simulink model "sampleModel1000"  (R2022a)
settings: Solver=VariableStepAuto  StartTime=0.0  StopTime=10.0  RelTol=1e-3
undefined symbols (not defined in the file): DiscIntNeverNeededParam, magnitude, Newton, Raphson
libraries: simulink x216, slpidlib x76
(part 2 of 10)

== system sampleModel1000/cfblk134 ==
  cfblk1 : Inport
  cfblk10 : Delay  SampleTime=1
  cfblk3 : simulink/Discrete/Transfer Fcn First Order  PoleZ=0.95  ICPrevOutput=0.0  DoSatur=off
  cfblk4 : DiscreteFir  SampleTime=1
  cfblk5 : slpidlib/PID Controller (2DOF)  Controller=PID  Form=Parallel  TimeDomain=Discrete-time  UseExternalTs=off  SampleTime=1  IntegratorMethod=Forward Euler  FilterMethod=Forward Euler  ControllerParametersSource=internal  P=1  I=1  UseKiTs=off  D=0  N=100  UseFilter=on  b=1  c=1  TunerSelectOption=Transfer Function Based (PID Tuner App)  InitialConditionSource=internal  InitialConditionForIntegrator=0  InitialConditionForFilter=0  DifferentiatorICPrevScaledInput=0  ExternalReset=none  TrackingMode=off  Kt=1  LimitOutput=off  SatLimitsSource=internal  UpperSaturationLimit=inf  LowerSaturationLimit=-inf  LinearizeAsGain=off  AntiWindupMode=none  Kb=1  POutMin=[]  POutMax=[]  IOutMin=[]  IOutMax=[]  DOutMin=[]  DOutMax=[]  NOutMin=[]  NOutMax=[]  bOutMin=[]  bOutMax=[]  cOutMin=[]  cOutMax=[]  SumOutMin=[]  SumOutMax=[]  SaturationOutMin=[]  SaturationOutMax=[]  PParamMin=[]  PParamMax=[]  IParamMin=[]  IParamMax=[]  DParamMin=[]  DParamMax=[]  NParamMin=[]  NParamMax=[]  bParamMin=[]  bParamMax=[]  cParamMin=[]  cParamMax=[]  KbParamMin=[]  KbParamMax=[]  KtParamMin=[]  KtParamMax=[]  KbOutMin=[]  KbOutMax=[]  KtOutMin=[]  KtOutMax=[]  IntegratorOutMin=[]  IntegratorOutMax=[]  FilterOutMin=[]  FilterOutMax=[]  SumI1OutMin=[]  SumI1OutMax=[]  SumI2OutMin=[]  SumI2OutMax=[]  SumI3OutMin=[]  SumI3OutMax=[]  SumI4OutMin=[]  SumI4OutMax=[]  SumDOutMin=[]  SumDOutMax=[]  Sum1OutMin=[]  Sum1OutMax=[]  Sum2OutMin=[]  Sum2OutMax=[]  Sum3OutMin=[]  Sum3OutMax=[]  DifferentiatorOutMin=[]  DifferentiatorOutMax=[]  FilterDiffOutCoefMin=[]  FilterDiffOutCoefMax=[]  ReciprocalOutMin=[]  ReciprocalOutMax=[]  SumDenOutMin=[]  SumDenOutMax=[]  SumNumOutMin=[]  SumNumOutMax=[]  DivideOutMin=[]  DivideOutMax=[]  UdiffTsProdOutMin=[]  UdiffTsProdOutMax=[]  NTsProdOutMin=[]  NTsProdOutMax=[]  UintegralTsProdOutMin=[]  UintegralTsProdOutMax=[]  UngainTsProdOutMin=[]  UngainTsProdOutMax=[]  IntegratorContinuousStateAttributes=''  IntegratorStateMustResolveToSignalObject=off  IntegratorRTWStateStorageClass=Auto  FilterContinuousStateAttributes=''  FilterStateMustResolveToSignalObject=off  FilterRTWStateStorageClass=Auto  ParallelPVariant=InternalParameters  IdealPVariant=Disabled  IVariant=InternalParameters  DVariant=InternalParameters  bVariant=InternalParameters  cVariant=InternalParameters  IntegratorVariant=Discrete  SatVariant=Disabled  AWVariant=Passthrough  PCopyVariant=Disabled  TRVariant=Disabled  FdbkBlocksVariant=Forward  IdealPFdbkVariant=Disabled  SatFdbkVariant=Disabled  DerivativeFilterVariant=ForwardEulerFilter  NVariant=InternalParameters  NCopyVariant=Disabled  FilterICVariant=InternalICsFilter  IntegratorICVariant=InternalICs  ExternalResetVariant=Disabled  TRSumVariant=Passthrough  SumFdbkVariant=Disabled  SumVariant=Sum_PID  TsampFilterVariant=InternalTs  TsampNgainVariant=Passthrough  TsampIntegralVariant=Passthrough  ExternalSaturationOutDataTypeStr=Inherit: Same as second input
      settings: SourceProductBaseCode=SL
  cfblk6 : DotProduct  OutDataTypeStr=Inherit: Inherit via internal rule
  cfblk7 : Product
  cfblk9 : Delay  SampleTime=1
  cfblk2 : Outport
  cfblk8 : Outport  Port=2
  wires:
  cfblk7/1 -> cfblk3/1, cfblk4/1
  cfblk5/1 -> cfblk6/1, cfblk2/1
  cfblk1/1 -> cfblk5/2
  cfblk6/1 -> cfblk7/1, cfblk7/2, cfblk8/1
  cfblk3/1 -> cfblk9/1
  cfblk9/1 -> cfblk5/1
  cfblk4/1 -> cfblk10/1
  cfblk10/1 -> cfblk6/2

== system sampleModel1000/cfblk135 ==
  cfblk1 : Inport
  cfblk15 : Inport  Port=2
  cfblk16 : Inport  Port=3
  cfblk10 : Sqrt
  cfblk11 : Constant  Value=[-838674796.182005]  SampleTime=1
  cfblk12 : Subsystem
  cfblk13 : Subsystem
  cfblk14 : Subsystem
  cfblk17 : Delay  SampleTime=1
  cfblk3 : DiscreteStateSpace
  cfblk4 : Delay  SampleTime=1
  cfblk5 : DiscreteZeroPole  Poles=[0 0.5]  Gain=1
  cfblk6 : Math  Operator=transpose
  cfblk7 : ComplexToRealImag
  cfblk8 : Product
  cfblk9 : simulink/Math Operations/Slider Gain  gain=1  low=0  high=2
  cfblk2 : Outport
  wires:
  cfblk5/1 -> cfblk3/1
  cfblk1/1 -> cfblk6/1
  cfblk11/1 -> cfblk14/1(cfblk1)
  cfblk15/1 -> cfblk10/1
  cfblk16/1 -> cfblk7/1
  cfblk8/1 -> cfblk12/1(cfblk1)
  cfblk12/1(cfblk2) -> cfblk9/1
  cfblk9/1 -> cfblk14/2(cfblk9)
  cfblk4/1 -> cfblk5/1
  cfblk7/1 -> cfblk14/3(cfblk10)
  cfblk13/1(cfblk2) -> cfblk4/1
  cfblk3/1 -> cfblk2/1
  cfblk10/1 -> cfblk8/2
  cfblk7/2 -> cfblk13/1(cfblk1)
  cfblk13/2(cfblk15) -> cfblk14/4(cfblk11)
  cfblk12/2(cfblk14) -> cfblk17/1
  cfblk17/1 -> cfblk8/1

== system sampleModel1000/cfblk136 ==
  cfblk1 : Inport
  cfblk9 : Inport  Port=2
  cfblk10 : Inport  Port=3
  cfblk12 : Delay  SampleTime=1
  cfblk13 : Delay  SampleTime=1
  cfblk3 : slpidlib/PID Controller  Controller=PID  Form=Parallel  TimeDomain=Discrete-time  UseExternalTs=off  SampleTime=1  IntegratorMethod=Forward Euler  FilterMethod=Forward Euler  ControllerParametersSource=internal  P=1  I=1  UseKiTs=off  D=0  N=100  UseFilter=on  TunerSelectOption=Transfer Function Based (PID Tuner App)  InitialConditionSource=internal  InitialConditionForIntegrator=0  InitialConditionForFilter=0  DifferentiatorICPrevScaledInput=0  ExternalReset=none  TrackingMode=off  Kt=1  LimitOutput=off  SatLimitsSource=internal  UpperSaturationLimit=inf  LowerSaturationLimit=-inf  LinearizeAsGain=off  AntiWindupMode=none  Kb=1  POutMin=[]  POutMax=[]  IOutMin=[]  IOutMax=[]  DOutMin=[]  DOutMax=[]  NOutMin=[]  NOutMax=[]  SumOutMin=[]  SumOutMax=[]  SaturationOutMin=[]  SaturationOutMax=[]  PParamMin=[]  PParamMax=[]  IParamMin=[]  IParamMax=[]  DParamMin=[]  DParamMax=[]  NParamMin=[]  NParamMax=[]  KbParamMin=[]  KbParamMax=[]  KtParamMin=[]  KtParamMax=[]  KbOutMin=[]  KbOutMax=[]  KtOutMin=[]  KtOutMax=[]  IntegratorOutMin=[]  IntegratorOutMax=[]  FilterOutMin=[]  FilterOutMax=[]  SumI1OutMin=[]  SumI1OutMax=[]  SumI2OutMin=[]  SumI2OutMax=[]  SumI3OutMin=[]  SumI3OutMax=[]  SumI4OutMin=[]  SumI4OutMax=[]  SumDOutMin=[]  SumDOutMax=[]  DifferentiatorOutMin=[]  DifferentiatorOutMax=[]  FilterDiffOutCoefMin=[]  FilterDiffOutCoefMax=[]  ReciprocalOutMin=[]  ReciprocalOutMax=[]  SumDenOutMin=[]  SumDenOutMax=[]  SumNumOutMin=[]  SumNumOutMax=[]  DivideOutMin=[]  DivideOutMax=[]  UdiffTsProdOutMin=[]  UdiffTsProdOutMax=[]  NTsProdOutMin=[]  NTsProdOutMax=[]  UintegralTsProdOutMin=[]  UintegralTsProdOutMax=[]  UngainTsProdOutMin=[]  UngainTsProdOutMax=[]  IntegratorContinuousStateAttributes=''  IntegratorStateMustResolveToSignalObject=off  IntegratorRTWStateStorageClass=Auto  FilterContinuousStateAttributes=''  FilterStateMustResolveToSignalObject=off  FilterRTWStateStorageClass=Auto  ParallelPVariant=InternalParameters  IdealPVariant=Disabled  IVariant=InternalParameters  DVariant=InternalParameters  IntegratorVariant=Discrete  SatVariant=Disabled  AWVariant=Passthrough  PCopyVariant=Disabled  TRVariant=Disabled  FdbkBlocksVariant=Forward  IdealPFdbkVariant=Disabled  SatFdbkVariant=Disabled  DerivativeFilterVariant=ForwardEulerFilter  NVariant=InternalParameters  NCopyVariant=Disabled  FilterICVariant=InternalICsFilter  IntegratorICVariant=InternalICs  ExternalResetVariant=Disabled  TRSumVariant=Passthrough  SumFdbkVariant=Disabled  SumVariant=Sum_PID  TsampFilterVariant=InternalTs  TsampNgainVariant=Passthrough  TsampIntegralVariant=Passthrough  ExternalSaturationOutDataTypeStr=Inherit: Same as second input  aMode=0
  cfblk4 : slpidlib/PID Controller  Controller=PID  Form=Parallel  TimeDomain=Discrete-time  UseExternalTs=off  SampleTime=1  IntegratorMethod=Forward Euler  FilterMethod=Forward Euler  ControllerParametersSource=internal  P=1  I=1  UseKiTs=off  D=0  N=100  UseFilter=on  TunerSelectOption=Transfer Function Based (PID Tuner App)  InitialConditionSource=internal  InitialConditionForIntegrator=0  InitialConditionForFilter=0  DifferentiatorICPrevScaledInput=0  ExternalReset=none  TrackingMode=off  Kt=1  LimitOutput=off  SatLimitsSource=internal  UpperSaturationLimit=inf  LowerSaturationLimit=-inf  LinearizeAsGain=off  AntiWindupMode=none  Kb=1  POutMin=[]  POutMax=[]  IOutMin=[]  IOutMax=[]  DOutMin=[]  DOutMax=[]  NOutMin=[]  NOutMax=[]  SumOutMin=[]  SumOutMax=[]  SaturationOutMin=[]  SaturationOutMax=[]  PParamMin=[]  PParamMax=[]  IParamMin=[]  IParamMax=[]  DParamMin=[]  DParamMax=[]  NParamMin=[]  NParamMax=[]  KbParamMin=[]  KbParamMax=[]  KtParamMin=[]  KtParamMax=[]  KbOutMin=[]  KbOutMax=[]  KtOutMin=[]  KtOutMax=[]  IntegratorOutMin=[]  IntegratorOutMax=[]  FilterOutMin=[]  FilterOutMax=[]  SumI1OutMin=[]  SumI1OutMax=[]  SumI2OutMin=[]  SumI2OutMax=[]  SumI3OutMin=[]  SumI3OutMax=[]  SumI4OutMin=[]  SumI4OutMax=[]  SumDOutMin=[]  SumDOutMax=[]  DifferentiatorOutMin=[]  DifferentiatorOutMax=[]  FilterDiffOutCoefMin=[]  FilterDiffOutCoefMax=[]  ReciprocalOutMin=[]  ReciprocalOutMax=[]  SumDenOutMin=[]  SumDenOutMax=[]  SumNumOutMin=[]  SumNumOutMax=[]  DivideOutMin=[]  DivideOutMax=[]  UdiffTsProdOutMin=[]  UdiffTsProdOutMax=[]  NTsProdOutMin=[]  NTsProdOutMax=[]  UintegralTsProdOutMin=[]  UintegralTsProdOutMax=[]  UngainTsProdOutMin=[]  UngainTsProdOutMax=[]  IntegratorContinuousStateAttributes=''  IntegratorStateMustResolveToSignalObject=off  IntegratorRTWStateStorageClass=Auto  FilterContinuousStateAttributes=''  FilterStateMustResolveToSignalObject=off  FilterRTWStateStorageClass=Auto  ParallelPVariant=InternalParameters  IdealPVariant=Disabled  IVariant=InternalParameters  DVariant=InternalParameters  IntegratorVariant=Discrete  SatVariant=Disabled  AWVariant=Passthrough  PCopyVariant=Disabled  TRVariant=Disabled  FdbkBlocksVariant=Forward  IdealPFdbkVariant=Disabled  SatFdbkVariant=Disabled  DerivativeFilterVariant=ForwardEulerFilter  NVariant=InternalParameters  NCopyVariant=Disabled  FilterICVariant=InternalICsFilter  IntegratorICVariant=InternalICs  ExternalResetVariant=Disabled  TRSumVariant=Passthrough  SumFdbkVariant=Disabled  SumVariant=Sum_PID  TsampFilterVariant=InternalTs  TsampNgainVariant=Passthrough  TsampIntegralVariant=Passthrough  ExternalSaturationOutDataTypeStr=Inherit: Same as second input  aMode=0
  cfblk5 : MinMax  Function=max  Inputs=2
  cfblk6 : Subsystem
  cfblk7 : Subsystem
  cfblk8 : Subsystem
  cfblk2 : Outport
  cfblk11 : Outport  Port=2
  wires:
  cfblk7/1(cfblk2) -> cfblk6/1(cfblk1)
  cfblk8/1(cfblk2) -> cfblk3/1
  cfblk10/1 -> cfblk4/1, cfblk8/4(cfblk9)
  cfblk8/2(cfblk12) -> cfblk2/1
  cfblk1/1 -> cfblk11/1, cfblk7/3(cfblk6)
  cfblk9/1 -> cfblk7/1(cfblk1)
  cfblk4/1 -> cfblk6/2(cfblk10)
  cfblk6/1(cfblk2) -> cfblk8/2(cfblk7), cfblk5/2, cfblk8/6(cfblk11)
  cfblk7/2(cfblk7) -> cfblk8/3(cfblk8), cfblk8/5(cfblk10)
  cfblk3/1 -> cfblk5/1, cfblk13/1
  cfblk5/1 -> cfblk12/1
  cfblk12/1 -> cfblk8/1(cfblk1)
  cfblk13/1 -> cfblk7/2(cfblk5)

== system sampleModel1000/cfblk137 ==
  cfblk1 : Inport
  cfblk13 : Inport  Port=2
  cfblk10 : Constant  Value=[-152590249.927515]  SampleTime=1
  cfblk11 : Constant  Value=[315107042.887950]  SampleTime=1
  cfblk12 : Subsystem
  cfblk3 : DiscreteFir  SampleTime=1
  cfblk4 : DiscreteStateSpace
  cfblk5 : Assignment  DiagnosticForDimensions=Warning  IndexOptions=Index vector (dialog)  Indices=1  OutputSizes=1
  cfblk6 : Sqrt  Operator=rSqrt  AlgorithmType=Newton-Raphson
  cfblk7 : Abs  SaturateOnIntegerOverflow=off
  cfblk8 : UnaryMinus
  cfblk9 : Signum
  cfblk2 : Outport
  cfblk14 : Outport  Port=2
  cfblk15 : Outport  Port=3
  wires:
  cfblk9/1 -> cfblk6/1
  cfblk13/1 -> cfblk12/1(cfblk1)
  cfblk8/1 -> cfblk5/1
  cfblk1/1 -> cfblk12/2(cfblk8)
  cfblk3/1 -> cfblk4/1
  cfblk4/1 -> cfblk2/1
  cfblk11/1 -> cfblk15/1
  cfblk10/1 -> cfblk7/1
  cfblk7/1 -> cfblk8/1
  cfblk6/1 -> cfblk5/2
  cfblk5/1 -> cfblk14/1
  cfblk12/1(cfblk2) -> cfblk3/1
  cfblk12/2(cfblk9) -> cfblk9/1

== system sampleModel1000/cfblk138 ==
  cfblk1 : Inport
  cfblk11 : Inport  Port=2
  cfblk10 : Subsystem
  cfblk3 : Delay  DelayLengthSource=Input port  SampleTime=1
      settings: InputPortMap=u0,p1
  cfblk4 : simulink/Discrete/Transfer Fcn Lead or Lag  PoleZ=0.95  ZeroZ=0.75  ICPrevOutput=0.0  ICPrevInput=0.0  DoSatur=off
      settings: SourceProductBaseCode=SL
  cfblk5 : ComplexToMagnitudeAngle
  cfblk6 : Trigonometry
  cfblk7 : Constant  Value=[211032908.922208]  SampleTime=1
  cfblk8 : Constant  Value=[325607232.572119]  SampleTime=1
  cfblk9 : Constant  Value=[286958174.606833]  SampleTime=1
  cfblk2 : Outport
  cfblk12 : Outport  Port=2
  wires:
  cfblk9/1 -> cfblk2/1
  cfblk10/1(cfblk2) -> cfblk12/1
  cfblk8/1 -> cfblk4/1
  cfblk11/1 -> cfblk3/1
  cfblk3/1 -> cfblk6/1
  cfblk5/1 -> cfblk3/2
  cfblk4/1 -> cfblk5/1
  cfblk7/1 -> cfblk10/1(cfblk1)
  cfblk1/1 -> cfblk10/2(cfblk13)
  cfblk6/1 -> cfblk10/3(cfblk14)

== system sampleModel1000/cfblk139 ==
  cfblk1 : Inport
  cfblk14 : Inport  Port=2
  cfblk15 : Inport  Port=3
  cfblk10 : Constant  Value=[730462996.486864]  SampleTime=1
  cfblk11 : Subsystem
  cfblk12 : Subsystem
  cfblk13 : Subsystem
  cfblk16 : Delay  SampleTime=1
  cfblk17 : Delay  SampleTime=1
  cfblk3 : slpidlib/PID Controller  Controller=PID  Form=Parallel  TimeDomain=Discrete-time  UseExternalTs=off  SampleTime=1  IntegratorMethod=Forward Euler  FilterMethod=Forward Euler  ControllerParametersSource=internal  P=1  I=1  UseKiTs=off  D=0  N=100  UseFilter=on  TunerSelectOption=Transfer Function Based (PID Tuner App)  InitialConditionSource=internal  InitialConditionForIntegrator=0  InitialConditionForFilter=0  DifferentiatorICPrevScaledInput=0  ExternalReset=none  TrackingMode=off  Kt=1  LimitOutput=off  SatLimitsSource=internal  UpperSaturationLimit=inf  LowerSaturationLimit=-inf  LinearizeAsGain=off  AntiWindupMode=none  Kb=1  POutMin=[]  POutMax=[]  IOutMin=[]  IOutMax=[]  DOutMin=[]  DOutMax=[]  NOutMin=[]  NOutMax=[]  SumOutMin=[]  SumOutMax=[]  SaturationOutMin=[]  SaturationOutMax=[]  PParamMin=[]  PParamMax=[]  IParamMin=[]  IParamMax=[]  DParamMin=[]  DParamMax=[]  NParamMin=[]  NParamMax=[]  KbParamMin=[]  KbParamMax=[]  KtParamMin=[]  KtParamMax=[]  KbOutMin=[]  KbOutMax=[]  KtOutMin=[]  KtOutMax=[]  IntegratorOutMin=[]  IntegratorOutMax=[]  FilterOutMin=[]  FilterOutMax=[]  SumI1OutMin=[]  SumI1OutMax=[]  SumI2OutMin=[]  SumI2OutMax=[]  SumI3OutMin=[]  SumI3OutMax=[]  SumI4OutMin=[]  SumI4OutMax=[]  SumDOutMin=[]  SumDOutMax=[]  DifferentiatorOutMin=[]  DifferentiatorOutMax=[]  FilterDiffOutCoefMin=[]  FilterDiffOutCoefMax=[]  ReciprocalOutMin=[]  ReciprocalOutMax=[]  SumDenOutMin=[]  SumDenOutMax=[]  SumNumOutMin=[]  SumNumOutMax=[]  DivideOutMin=[]  DivideOutMax=[]  UdiffTsProdOutMin=[]  UdiffTsProdOutMax=[]  NTsProdOutMin=[]  NTsProdOutMax=[]  UintegralTsProdOutMin=[]  UintegralTsProdOutMax=[]  UngainTsProdOutMin=[]  UngainTsProdOutMax=[]  IntegratorContinuousStateAttributes=''  IntegratorStateMustResolveToSignalObject=off  IntegratorRTWStateStorageClass=Auto  FilterContinuousStateAttributes=''  FilterStateMustResolveToSignalObject=off  FilterRTWStateStorageClass=Auto  ParallelPVariant=InternalParameters  IdealPVariant=Disabled  IVariant=InternalParameters  DVariant=InternalParameters  IntegratorVariant=Discrete  SatVariant=Disabled  AWVariant=Passthrough  PCopyVariant=Disabled  TRVariant=Disabled  FdbkBlocksVariant=Forward  IdealPFdbkVariant=Disabled  SatFdbkVariant=Disabled  DerivativeFilterVariant=ForwardEulerFilter  NVariant=InternalParameters  NCopyVariant=Disabled  FilterICVariant=InternalICsFilter  IntegratorICVariant=InternalICs  ExternalResetVariant=Disabled  TRSumVariant=Passthrough  SumFdbkVariant=Disabled  SumVariant=Sum_PID  TsampFilterVariant=InternalTs  TsampNgainVariant=Passthrough  TsampIntegralVariant=Passthrough  ExternalSaturationOutDataTypeStr=Inherit: Same as second input  aMode=0
  cfblk4 : DiscreteTransferFcn  SampleTime=1
  cfblk5 : UnitDelay  HasFrameUpgradeWarning=on
  cfblk6 : simulink/Math Operations/MinMax Running Resettable  Function=min  vinit=0.0
  cfblk7 : PermuteDimensions
  cfblk8 : UnaryMinus
  cfblk9 : MinMax  Inputs=3
  cfblk2 : Outport
  wires:
  cfblk3/1 -> cfblk5/1
  cfblk9/1 -> cfblk7/1
  cfblk7/1 -> cfblk6/1
  cfblk8/1 -> cfblk9/1
  cfblk4/1 -> cfblk12/1(cfblk1)
  cfblk14/1 -> cfblk9/2, cfblk11/3(cfblk10)
  cfblk5/1 -> cfblk12/2(cfblk10), cfblk4/1
  cfblk10/1 -> cfblk3/1
  cfblk12/1(cfblk2) -> cfblk8/1
  cfblk15/1 -> cfblk11/1(cfblk1)
  cfblk1/1 -> cfblk12/3(cfblk11), cfblk13/2(cfblk10), cfblk12/4(cfblk12), cfblk13/3(cfblk11), cfblk11/4(cfblk11)
  cfblk13/1(cfblk2) -> cfblk11/2(cfblk9), cfblk12/5(cfblk13)
  cfblk12/2(cfblk14) -> cfblk6/2
  cfblk12/3(cfblk15) -> cfblk2/1
  cfblk6/1 -> cfblk16/1
  cfblk16/1 -> cfblk9/3
  cfblk11/1(cfblk2) -> cfblk17/1
  cfblk17/1 -> cfblk13/1(cfblk1)

== system sampleModel1000/cfblk140 ==
  cfblk1 : Inport
  cfblk8 : Inport  Port=2
  cfblk{9..13} (5 alike) : Delay  SampleTime=1
  cfblk3 : simulink/Discrete/Transfer Fcn Real Zero  ZeroZ=0.75  ICPrevInput=0.0  DoSatur=off
      settings: SourceProductBaseCode=SL
  cfblk4 : Delay  DelayLengthSource=Input port  SampleTime=1
      settings: InputPortMap=u0,p1
  cfblk5 : UnitDelay  HasFrameUpgradeWarning=on
  cfblk6 : Subsystem
  cfblk7 : Subsystem
  cfblk2 : Outport
  wires:
  cfblk5/1 -> cfblk6/1(cfblk1)
  cfblk8/1 -> cfblk5/1
  cfblk1/1 -> cfblk7/2(cfblk15), cfblk4/2
  cfblk6/1(cfblk2) -> cfblk3/1
  cfblk3/1 -> cfblk2/1, cfblk4/1, cfblk10/1, cfblk11/1, cfblk12/1
  cfblk7/1(cfblk2) -> cfblk6/2(cfblk8)
  cfblk4/1 -> cfblk9/1
  cfblk9/1 -> cfblk7/1(cfblk1)
  cfblk10/1 -> cfblk6/3(cfblk9)
  cfblk11/1 -> cfblk6/4(cfblk10)
  cfblk12/1 -> cfblk7/4(cfblk17)
  cfblk6/2(cfblk11) -> cfblk13/1
  cfblk13/1 -> cfblk7/3(cfblk16)

== system sampleModel1000/cfblk141 ==
  cfblk1 : Inport
  cfblk9 : Inport  Port=2
  cfblk10 : Inport  Port=3
  cfblk11 : Inport  Port=4
  cfblk3 : Delay  SampleTime=1
  cfblk4 : DiscreteZeroPole  Poles=[0 0.5]  Gain=1
  cfblk5 : Sin  TimeSource=Use external signal  SampleTime=0
  cfblk6 : Reshape
  cfblk7 : Product  Inputs=*
  cfblk8 : Subsystem
  cfblk2 : Outport
  wires:
  cfblk11/1 -> cfblk3/1
  cfblk6/1 -> cfblk4/1
  cfblk3/1 -> cfblk6/1
  cfblk7/1 -> cfblk5/1
  cfblk5/1 -> cfblk8/1(cfblk1)
  cfblk4/1 -> cfblk7/1
  cfblk9/1 -> cfblk8/2(cfblk12)
  cfblk10/1 -> cfblk8/3(cfblk13)
  cfblk8/1(cfblk2) -> cfblk2/1

== system sampleModel1000/cfblk142 ==
  cfblk1 : Inport
  cfblk10 : Subsystem
  cfblk11 : Subsystem
  cfblk12 : Subsystem
  cfblk13 : Subsystem
  cfblk{15..18} (4 alike) : Delay  SampleTime=1
  cfblk3 : DiscreteFir  SampleTime=1
  cfblk4 : simulink/Discrete/Transfer Fcn Lead or Lag  PoleZ=0.95  ZeroZ=0.75  ICPrevOutput=0.0  ICPrevInput=0.0  DoSatur=off
      settings: SourceProductBaseCode=SL
  cfblk5 : ComplexToMagnitudeAngle
  cfblk6 : Product  Inputs=**
  cfblk7 : ComplexToMagnitudeAngle
  cfblk8 : Product  Inputs=*
  cfblk9 : Constant  Value=[148580806.224860]  SampleTime=1
  cfblk2 : Outport
  cfblk14 : Outport  Port=2
  wires:
  cfblk1/1 -> cfblk10/1(cfblk1)
  cfblk6/1 -> cfblk13/3(cfblk14), cfblk18/1
  cfblk7/1 -> cfblk4/1
  cfblk10/1(cfblk2) -> cfblk8/1
  cfblk8/1 -> cfblk7/1, cfblk13/2(cfblk13)
  cfblk9/1 -> cfblk6/1
  cfblk12/1(cfblk2) -> cfblk5/1
  cfblk10/2(cfblk12) -> cfblk13/1(cfblk1), cfblk12/4(cfblk9)
  cfblk11/1(cfblk2) -> cfblk3/1
  cfblk3/1 -> cfblk15/1, cfblk16/1
  cfblk4/1 -> cfblk14/1, cfblk11/4(cfblk15)
  cfblk13/1(cfblk2) -> cfblk2/1
  cfblk7/2 -> cfblk11/2(cfblk13)
  cfblk5/2 -> cfblk6/2
  cfblk11/2(cfblk16) -> cfblk12/2(cfblk7)
  cfblk11/3(cfblk17) -> cfblk12/3(cfblk8)
  cfblk15/1 -> cfblk11/1(cfblk1)
  cfblk16/1 -> cfblk11/3(cfblk14)
  cfblk5/1 -> cfblk17/1
  cfblk17/1 -> cfblk12/1(cfblk1)
  cfblk18/1 -> cfblk10/2(cfblk11)

== system sampleModel1000/cfblk143 ==
  cfblk1 : Inport
  cfblk12 : Inport  Port=2
  cfblk10 : Constant  Value=[905866225.298065]  SampleTime=1
  cfblk11 : Subsystem
  cfblk14 : Delay  SampleTime=1
  cfblk3 : Abs  SaturateOnIntegerOverflow=off
  cfblk4 : Rounding
  cfblk5 : Sqrt  Operator=rSqrt  AlgorithmType=Newton-Raphson
  cfblk6 : Sum  Inputs=-+
  cfblk7 : Abs  SaturateOnIntegerOverflow=off
  cfblk8 : Sum  Inputs=+-
  cfblk9 : Constant  Value=[459060149.907178]  SampleTime=1
  cfblk2 : Outport
  cfblk13 : Outport  Port=2
  wires:
  cfblk1/1 -> cfblk2/1
  cfblk6/1 -> cfblk11/1(cfblk1)
  cfblk9/1 -> cfblk4/1
  cfblk7/1 -> cfblk6/1
  cfblk5/1 -> cfblk8/1
  cfblk3/1 -> cfblk7/1
  cfblk10/1 -> cfblk8/2, cfblk11/3(cfblk10)
  cfblk12/1 -> cfblk3/1
  cfblk8/1 -> cfblk13/1, cfblk14/1
  cfblk4/1 -> cfblk6/2
  cfblk11/1(cfblk2) -> cfblk5/1
  cfblk14/1 -> cfblk11/2(cfblk9)

== system sampleModel1000/cfblk144 ==
  cfblk1 : Inport
  cfblk7 : Inport  Port=2
  cfblk8 : Inport  Port=3
  cfblk3 : slpidlib/PID Controller  Controller=PID  Form=Parallel  TimeDomain=Discrete-time  UseExternalTs=off  SampleTime=1  IntegratorMethod=Forward Euler  FilterMethod=Forward Euler  ControllerParametersSource=internal  P=1  I=1  UseKiTs=off  D=0  N=100  UseFilter=on  TunerSelectOption=Transfer Function Based (PID Tuner App)  InitialConditionSource=internal  InitialConditionForIntegrator=0  InitialConditionForFilter=0  DifferentiatorICPrevScaledInput=0  ExternalReset=none  TrackingMode=off  Kt=1  LimitOutput=off  SatLimitsSource=internal  UpperSaturationLimit=inf  LowerSaturationLimit=-inf  LinearizeAsGain=off  AntiWindupMode=none  Kb=1  POutMin=[]  POutMax=[]  IOutMin=[]  IOutMax=[]  DOutMin=[]  DOutMax=[]  NOutMin=[]  NOutMax=[]  SumOutMin=[]  SumOutMax=[]  SaturationOutMin=[]  SaturationOutMax=[]  PParamMin=[]  PParamMax=[]  IParamMin=[]  IParamMax=[]  DParamMin=[]  DParamMax=[]  NParamMin=[]  NParamMax=[]  KbParamMin=[]  KbParamMax=[]  KtParamMin=[]  KtParamMax=[]  KbOutMin=[]  KbOutMax=[]  KtOutMin=[]  KtOutMax=[]  IntegratorOutMin=[]  IntegratorOutMax=[]  FilterOutMin=[]  FilterOutMax=[]  SumI1OutMin=[]  SumI1OutMax=[]  SumI2OutMin=[]  SumI2OutMax=[]  SumI3OutMin=[]  SumI3OutMax=[]  SumI4OutMin=[]  SumI4OutMax=[]  SumDOutMin=[]  SumDOutMax=[]  DifferentiatorOutMin=[]  DifferentiatorOutMax=[]  FilterDiffOutCoefMin=[]  FilterDiffOutCoefMax=[]  ReciprocalOutMin=[]  ReciprocalOutMax=[]  SumDenOutMin=[]  SumDenOutMax=[]  SumNumOutMin=[]  SumNumOutMax=[]  DivideOutMin=[]  DivideOutMax=[]  UdiffTsProdOutMin=[]  UdiffTsProdOutMax=[]  NTsProdOutMin=[]  NTsProdOutMax=[]  UintegralTsProdOutMin=[]  UintegralTsProdOutMax=[]  UngainTsProdOutMin=[]  UngainTsProdOutMax=[]  IntegratorContinuousStateAttributes=''  IntegratorStateMustResolveToSignalObject=off  IntegratorRTWStateStorageClass=Auto  FilterContinuousStateAttributes=''  FilterStateMustResolveToSignalObject=off  FilterRTWStateStorageClass=Auto  ParallelPVariant=InternalParameters  IdealPVariant=Disabled  IVariant=InternalParameters  DVariant=InternalParameters  IntegratorVariant=Discrete  SatVariant=Disabled  AWVariant=Passthrough  PCopyVariant=Disabled  TRVariant=Disabled  FdbkBlocksVariant=Forward  IdealPFdbkVariant=Disabled  SatFdbkVariant=Disabled  DerivativeFilterVariant=ForwardEulerFilter  NVariant=InternalParameters  NCopyVariant=Disabled  FilterICVariant=InternalICsFilter  IntegratorICVariant=InternalICs  ExternalResetVariant=Disabled  TRSumVariant=Passthrough  SumFdbkVariant=Disabled  SumVariant=Sum_PID  TsampFilterVariant=InternalTs  TsampNgainVariant=Passthrough  TsampIntegralVariant=Passthrough  ExternalSaturationOutDataTypeStr=Inherit: Same as second input  aMode=0
  cfblk4 : Delay  DelayLengthSource=Input port  SampleTime=1
      settings: InputPortMap=u0,p1
  cfblk5 : Gain  Gain=[419845500.922329]
  cfblk6 : Subsystem
  cfblk2 : Outport
  cfblk9 : Outport  Port=2
  wires:
  cfblk6/1(cfblk2) -> cfblk3/1
  cfblk1/1 -> cfblk5/1, cfblk6/4(cfblk14)
  cfblk3/1 -> cfblk2/1
  cfblk5/1 -> cfblk4/1, cfblk4/2, cfblk9/1
  cfblk8/1 -> cfblk6/1(cfblk1), cfblk6/5(cfblk15), cfblk6/6(cfblk16)
  cfblk7/1 -> cfblk6/2(cfblk12)
  cfblk4/1 -> cfblk6/3(cfblk13)

== system sampleModel1000/cfblk145 ==
  cfblk1 : Inport
  cfblk12 : Inport  Port=2
  cfblk13 : Inport  Port=3
  cfblk10 : Subsystem
  cfblk11 : Subsystem
  cfblk{16..19} (4 alike) : Delay  SampleTime=1
  cfblk3 : DiscreteStateSpace
  cfblk4 : ComplexToRealImag
  cfblk5 : Constant  Value=[-195042081.947706]  SampleTime=1
  cfblk6 : Constant  Value=[-214759088.337772]  SampleTime=1
  cfblk7 : Subsystem
  cfblk8 : Subsystem
  cfblk9 : Subsystem
  cfblk2 : Outport
  cfblk14 : Outport  Port=2
  cfblk15 : Outport  Port=3
  wires:
  cfblk9/1(cfblk2) -> cfblk2/1
  cfblk12/1 -> cfblk8/1(cfblk1)
  cfblk4/1 -> cfblk3/1
  cfblk9/2(cfblk12) -> cfblk8/2(cfblk7)
  cfblk13/1 -> cfblk15/1, cfblk7/5(cfblk15)
  cfblk7/1(cfblk2) -> cfblk14/1
  cfblk8/1(cfblk2) -> cfblk11/1(cfblk1)
  cfblk4/2 -> cfblk10/1(cfblk1)
  cfblk1/1 -> cfblk7/1(cfblk1), cfblk7/4(cfblk14), cfblk7/6(cfblk16)
  cfblk5/1 -> cfblk8/3(cfblk8)
  cfblk7/2(cfblk17) -> cfblk9/1(cfblk1)
  cfblk6/1 -> cfblk4/1
  cfblk3/1 -> cfblk10/2(cfblk16)
  cfblk8/2(cfblk9) -> cfblk10/3(cfblk17)
  cfblk11/1(cfblk2) -> cfblk16/1
  cfblk16/1 -> cfblk9/2(cfblk10)
  cfblk11/2(cfblk6) -> cfblk17/1
  cfblk17/1 -> cfblk7/2(cfblk12)
  cfblk11/3(cfblk7) -> cfblk18/1
  cfblk18/1 -> cfblk7/3(cfblk13)
  cfblk10/1(cfblk2) -> cfblk19/1
  cfblk19/1 -> cfblk9/3(cfblk11)

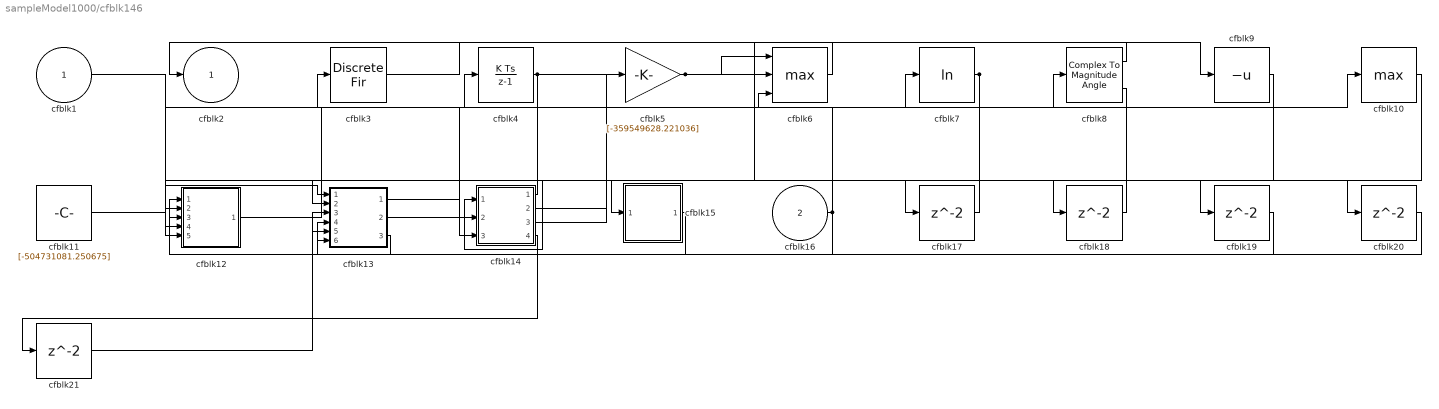
== system sampleModel1000/cfblk146 ==
  cfblk1 : Inport
  cfblk16 : Inport  Port=2
  cfblk10 : MinMax  Function=max
  cfblk11 : Constant  Value=[-504731081.250675]  SampleTime=1
  cfblk12 : Subsystem
  cfblk13 : Subsystem
  cfblk14 : Subsystem
  cfblk15 : Subsystem
  cfblk{17..21} (5 alike) : Delay  SampleTime=1
  cfblk3 : DiscreteFir  SampleTime=1
  cfblk4 : DiscreteIntegrator  ICPrevOutput=DiscIntNeverNeededParam  ICPrevScaledInput=DiscIntNeverNeededParam
  cfblk5 : Gain  Gain=[-359549628.221036]
  cfblk6 : MinMax  Function=max  Inputs=3
  cfblk7 : Math  Operator=log
  cfblk8 : ComplexToMagnitudeAngle
  cfblk9 : UnaryMinus
  cfblk2 : Outport
  wires:
  cfblk14/1(cfblk2) -> cfblk4/1
  cfblk6/1 -> cfblk2/1
  cfblk15/1(cfblk2) -> cfblk12/1(cfblk1)
  cfblk7/1 -> cfblk14/1(cfblk1), cfblk12/4(cfblk15)
  cfblk9/1 -> cfblk15/1(cfblk1)
  cfblk14/2(cfblk14) -> cfblk10/1
  cfblk10/1 -> cfblk12/2(cfblk13)
  cfblk5/1 -> cfblk6/1, cfblk19/1, cfblk20/1
  cfblk3/1 -> cfblk9/1
  cfblk12/1(cfblk2) -> cfblk8/1
  cfblk4/1 -> cfblk12/5(cfblk16), cfblk17/1
  cfblk1/1 -> cfblk13/1(cfblk1)
  cfblk16/1 -> cfblk3/1, cfblk13/4(cfblk13)
  cfblk8/1 -> cfblk6/2
  cfblk11/1 -> cfblk7/1
  cfblk13/1(cfblk2) -> cfblk6/3
  cfblk14/3(cfblk15) -> cfblk5/1
  cfblk13/2(cfblk16) -> cfblk14/3(cfblk13)
  cfblk13/3(cfblk17) -> cfblk12/3(cfblk14)
  cfblk17/1 -> cfblk14/2(cfblk12)
  cfblk8/2 -> cfblk18/1
  cfblk18/1 -> cfblk13/2(cfblk11)
  cfblk19/1 -> cfblk13/5(cfblk14)
  cfblk20/1 -> cfblk13/6(cfblk15)
  cfblk14/4(cfblk16) -> cfblk21/1
  cfblk21/1 -> cfblk13/3(cfblk12)

== system sampleModel1000/cfblk147 ==
  cfblk1 : Inport
  cfblk12 : Inport  Port=2
  cfblk10 : Subsystem
  cfblk11 : Subsystem
  cfblk{13..16} (4 alike) : Delay  SampleTime=1
  cfblk3 : DiscreteTransferFcn  SampleTime=1
  cfblk4 : Gain  Gain=[54054691.102127]
  cfblk5 : Reshape
  cfblk6 : PermuteDimensions
  cfblk7 : Subsystem
  cfblk8 : Subsystem
  cfblk9 : Subsystem
  cfblk2 : Outport
  wires:
  cfblk8/1(cfblk2) -> cfblk10/1(cfblk1)
  cfblk9/1(cfblk2) -> cfblk11/1(cfblk1)
  cfblk5/1 -> cfblk8/1(cfblk1)
  cfblk11/1(cfblk2) -> cfblk3/1
  cfblk11/2(cfblk12) -> cfblk10/2(cfblk14)
  cfblk9/2(cfblk7) -> cfblk5/1
  cfblk1/1 -> cfblk6/1
  cfblk12/1 -> cfblk10/3(cfblk15)
  cfblk6/1 -> cfblk7/3(cfblk11), cfblk11/2(cfblk11)
  cfblk11/3(cfblk13) -> cfblk8/2(cfblk11), cfblk10/5(cfblk17)
  cfblk7/1(cfblk2) -> cfblk9/3(cfblk6), cfblk4/1
  cfblk4/1 -> cfblk2/1, cfblk10/4(cfblk16)
  cfblk3/1 -> cfblk13/1
  cfblk13/1 -> cfblk7/1(cfblk1)
  cfblk10/1(cfblk2) -> cfblk14/1
  cfblk14/1 -> cfblk7/2(cfblk10)
  cfblk8/2(cfblk12) -> cfblk15/1
  cfblk15/1 -> cfblk9/1(cfblk1)
  cfblk8/3(cfblk13) -> cfblk16/1
  cfblk16/1 -> cfblk9/2(cfblk5)

== system sampleModel1000/cfblk148 ==
  cfblk1 : Inport
  cfblk3 : DiscreteStateSpace
  cfblk4 : Math  Operator=10^u
  cfblk5 : Subsystem
  cfblk6 : Subsystem
  cfblk8 : Delay  SampleTime=1
  cfblk9 : Delay  SampleTime=1
  cfblk2 : Outport
  cfblk7 : Outport  Port=2
  wires:
  cfblk5/1(cfblk2) -> cfblk4/1
  cfblk4/1 -> cfblk6/1(cfblk1), cfblk8/1
  cfblk5/2(cfblk16) -> cfblk3/1
  cfblk1/1 -> cfblk5/2(cfblk14), cfblk6/2(cfblk14), cfblk6/3(cfblk15), cfblk6/4(cfblk16)
  cfblk6/1(cfblk2) -> cfblk7/1
  cfblk5/3(cfblk17) -> cfblk2/1
  cfblk8/1 -> cfblk5/1(cfblk1)
  cfblk3/1 -> cfblk9/1
  cfblk9/1 -> cfblk5/3(cfblk15)

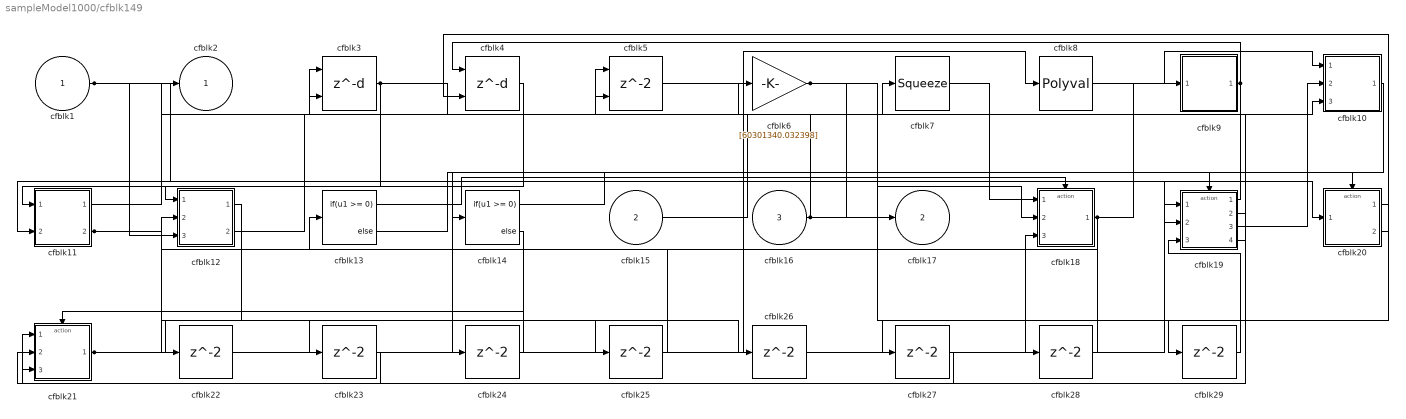
== system sampleModel1000/cfblk149 ==
  cfblk1 : Inport
  cfblk15 : Inport  Port=2
  cfblk16 : Inport  Port=3
  cfblk10 : Subsystem
  cfblk11 : Subsystem
  cfblk12 : Subsystem
  cfblk13 : If  IfExpression=u1 >= 0  SampleTime=1
  cfblk14 : If  IfExpression=u1 >= 0  SampleTime=1
  cfblk18 : Subsystem  TreatAsAtomicUnit=on
  cfblk19 : Subsystem  TreatAsAtomicUnit=on
  cfblk20 : Subsystem  TreatAsAtomicUnit=on
  cfblk21 : Subsystem  TreatAsAtomicUnit=on
  cfblk{22..29} (8 alike) : Delay  SampleTime=1
  cfblk3 : Delay  DelayLengthSource=Input port  SampleTime=1
      settings: InputPortMap=u0,p1
  cfblk4 : Delay  DelayLengthSource=Input port  SampleTime=1
      settings: InputPortMap=u0,p1
  cfblk5 : Delay  ShowEnablePort=on  SampleTime=1
      settings: InputPortMap=u0,e6
  cfblk6 : Gain  Gain=[60301340.032398]
  cfblk7 : Squeeze
  cfblk8 : Polyval  Coefs=[ +2.081618890e-019, -1.441693666e-014, +4.719686976e-010, -8.536869453e-006, +1.621573104e-001, -8.087801117e+001 ]
  cfblk9 : Subsystem
  cfblk2 : Outport
  cfblk17 : Outport  Port=2
  wires:
  cfblk6/1 -> cfblk17/1, cfblk29/1
  cfblk7/1 -> cfblk18/1(cfblk1)
  cfblk18/1(cfblk2) -> cfblk9/1(cfblk1), cfblk27/1
  cfblk21/1(cfblk2) -> cfblk8/1, cfblk25/1
  cfblk16/1 -> cfblk3/1, cfblk18/2(cfblk15)
  cfblk9/1(cfblk2) -> cfblk4/1, cfblk11/2(cfblk8)
  cfblk15/1 -> cfblk7/1
  cfblk5/1 -> cfblk20/1(cfblk1)
  cfblk8/1 -> cfblk10/1(cfblk1)
  cfblk12/2(cfblk14) -> cfblk5/1
  cfblk4/1 -> cfblk11/1(cfblk1)
  cfblk20/2(cfblk13) -> cfblk4/2
  cfblk19/1(cfblk2) -> cfblk3/2
  cfblk3/1 -> cfblk12/1(cfblk1), cfblk10/3(cfblk14)
  cfblk1/1 -> cfblk19/2(cfblk13), cfblk5/2, cfblk12/3(cfblk13)
  cfblk11/1(cfblk2) -> cfblk2/1
  cfblk19/2(cfblk15) -> cfblk21/1(cfblk1)
  cfblk11/2(cfblk9) -> cfblk23/1, cfblk26/1
  cfblk19/3(cfblk16) -> cfblk10/2(cfblk13)
  cfblk19/4(cfblk17) -> cfblk6/1
  cfblk13/1 -> cfblk18/Action
  cfblk13/2 -> cfblk19/Action
  cfblk14/1 -> cfblk20/Action
  cfblk14/2 -> cfblk21/Action
  cfblk12/1(cfblk2) -> cfblk22/1
  cfblk22/1 -> cfblk19/1(cfblk1)
  cfblk23/1 -> cfblk21/2(cfblk16)
  cfblk10/1(cfblk2) -> cfblk24/1
  cfblk24/1 -> cfblk14/1
  cfblk25/1 -> cfblk12/2(cfblk12)
  cfblk26/1 -> cfblk18/3(cfblk16)
  cfblk27/1 -> cfblk21/3(cfblk17)
  cfblk20/1(cfblk2) -> cfblk28/1
  cfblk28/1 -> cfblk13/1
  cfblk29/1 -> cfblk19/3(cfblk14)

== system sampleModel1000/cfblk150 ==
  cfblk1 : Inport
  cfblk11 : Inport  Port=2
  cfblk10 : Subsystem
  cfblk{3,12..19} (9 alike) : Delay  SampleTime=1
  cfblk4 : slpidlib/PID Controller (2DOF)  Controller=PID  Form=Parallel  TimeDomain=Discrete-time  UseExternalTs=off  SampleTime=1  IntegratorMethod=Forward Euler  FilterMethod=Forward Euler  ControllerParametersSource=internal  P=1  I=1  UseKiTs=off  D=0  N=100  UseFilter=on  b=1  c=1  TunerSelectOption=Transfer Function Based (PID Tuner App)  InitialConditionSource=internal  InitialConditionForIntegrator=0  InitialConditionForFilter=0  DifferentiatorICPrevScaledInput=0  ExternalReset=none  TrackingMode=off  Kt=1  LimitOutput=off  SatLimitsSource=internal  UpperSaturationLimit=inf  LowerSaturationLimit=-inf  LinearizeAsGain=off  AntiWindupMode=none  Kb=1  POutMin=[]  POutMax=[]  IOutMin=[]  IOutMax=[]  DOutMin=[]  DOutMax=[]  NOutMin=[]  NOutMax=[]  bOutMin=[]  bOutMax=[]  cOutMin=[]  cOutMax=[]  SumOutMin=[]  SumOutMax=[]  SaturationOutMin=[]  SaturationOutMax=[]  PParamMin=[]  PParamMax=[]  IParamMin=[]  IParamMax=[]  DParamMin=[]  DParamMax=[]  NParamMin=[]  NParamMax=[]  bParamMin=[]  bParamMax=[]  cParamMin=[]  cParamMax=[]  KbParamMin=[]  KbParamMax=[]  KtParamMin=[]  KtParamMax=[]  KbOutMin=[]  KbOutMax=[]  KtOutMin=[]  KtOutMax=[]  IntegratorOutMin=[]  IntegratorOutMax=[]  FilterOutMin=[]  FilterOutMax=[]  SumI1OutMin=[]  SumI1OutMax=[]  SumI2OutMin=[]  SumI2OutMax=[]  SumI3OutMin=[]  SumI3OutMax=[]  SumI4OutMin=[]  SumI4OutMax=[]  SumDOutMin=[]  SumDOutMax=[]  Sum1OutMin=[]  Sum1OutMax=[]  Sum2OutMin=[]  Sum2OutMax=[]  Sum3OutMin=[]  Sum3OutMax=[]  DifferentiatorOutMin=[]  DifferentiatorOutMax=[]  FilterDiffOutCoefMin=[]  FilterDiffOutCoefMax=[]  ReciprocalOutMin=[]  ReciprocalOutMax=[]  SumDenOutMin=[]  SumDenOutMax=[]  SumNumOutMin=[]  SumNumOutMax=[]  DivideOutMin=[]  DivideOutMax=[]  UdiffTsProdOutMin=[]  UdiffTsProdOutMax=[]  NTsProdOutMin=[]  NTsProdOutMax=[]  UintegralTsProdOutMin=[]  UintegralTsProdOutMax=[]  UngainTsProdOutMin=[]  UngainTsProdOutMax=[]  IntegratorContinuousStateAttributes=''  IntegratorStateMustResolveToSignalObject=off  IntegratorRTWStateStorageClass=Auto  FilterContinuousStateAttributes=''  FilterStateMustResolveToSignalObject=off  FilterRTWStateStorageClass=Auto  ParallelPVariant=InternalParameters  IdealPVariant=Disabled  IVariant=InternalParameters  DVariant=InternalParameters  bVariant=InternalParameters  cVariant=InternalParameters  IntegratorVariant=Discrete  SatVariant=Disabled  AWVariant=Passthrough  PCopyVariant=Disabled  TRVariant=Disabled  FdbkBlocksVariant=Forward  IdealPFdbkVariant=Disabled  SatFdbkVariant=Disabled  DerivativeFilterVariant=ForwardEulerFilter  NVariant=InternalParameters  NCopyVariant=Disabled  FilterICVariant=InternalICsFilter  IntegratorICVariant=InternalICs  ExternalResetVariant=Disabled  TRSumVariant=Passthrough  SumFdbkVariant=Disabled  SumVariant=Sum_PID  TsampFilterVariant=InternalTs  TsampNgainVariant=Passthrough  TsampIntegralVariant=Passthrough  ExternalSaturationOutDataTypeStr=Inherit: Same as second input
      settings: SourceProductBaseCode=SL
  cfblk5 : Bias  Bias=[-365167928.627843]  SaturateOnIntegerOverflow=off
  cfblk6 : Product  Inputs=**
  cfblk7 : Subsystem
  cfblk8 : Subsystem
  cfblk9 : Subsystem
  cfblk2 : Outport
  wires:
  cfblk6/1 -> cfblk4/1, cfblk9/4(cfblk16), cfblk16/1
  cfblk11/1 -> cfblk2/1
  cfblk4/1 -> cfblk5/1
  cfblk7/1(cfblk2) -> cfblk8/1(cfblk1)
  cfblk1/1 -> cfblk10/1(cfblk1), cfblk4/2, cfblk9/5(cfblk17), cfblk6/2
  cfblk5/1 -> cfblk9/1(cfblk1)
  cfblk3/1 -> cfblk9/2(cfblk14), cfblk18/1
  cfblk9/1(cfblk2) -> cfblk13/1, cfblk14/1, cfblk15/1
  cfblk7/2(cfblk10) -> cfblk9/3(cfblk15), cfblk3/1, cfblk19/1
  cfblk8/1(cfblk2) -> cfblk6/1, cfblk12/1, cfblk17/1
  cfblk10/1(cfblk2) -> cfblk7/1(cfblk1)
  cfblk10/2(cfblk15) -> cfblk8/3(cfblk16)
  cfblk10/3(cfblk16) -> cfblk8/4(cfblk17)
  cfblk12/1 -> cfblk10/2(cfblk11)
  cfblk13/1 -> cfblk8/2(cfblk15)
  cfblk14/1 -> cfblk7/3(cfblk8)
  cfblk15/1 -> cfblk10/5(cfblk14)
  cfblk16/1 -> cfblk10/3(cfblk12)
  cfblk17/1 -> cfblk7/2(cfblk7)
  cfblk18/1 -> cfblk7/4(cfblk9)
  cfblk19/1 -> cfblk10/4(cfblk13)

== system sampleModel1000/cfblk151 ==
  cfblk1 : Inport
  cfblk6 : Inport  Port=2
  cfblk7 : Inport  Port=3
  cfblk3 : DiscreteFir  SampleTime=1
  cfblk4 : Subsystem
  cfblk5 : Subsystem
  cfblk8 : Delay  SampleTime=1
  cfblk2 : Outport
  wires:
  cfblk1/1 -> cfblk5/1(cfblk1)
  cfblk7/1 -> cfblk4/1(cfblk1)
  cfblk6/1 -> cfblk3/1
  cfblk5/1(cfblk2) -> cfblk2/1, cfblk4/3(cfblk9)
  cfblk3/1 -> cfblk4/2(cfblk8)
  cfblk4/1(cfblk2) -> cfblk8/1
  cfblk8/1 -> cfblk5/2(cfblk10)

== system sampleModel1000/cfblk152 ==
  cfblk1 : Inport
  cfblk10 : Delay  SampleTime=1
  cfblk3 : Sqrt  Operator=rSqrt  AlgorithmType=Newton-Raphson
  cfblk4 : DotProduct  OutDataTypeStr=Inherit: Inherit via internal rule
  cfblk5 : Subsystem
  cfblk6 : Subsystem
  cfblk8 : Delay  SampleTime=1
  cfblk9 : Delay  SampleTime=1
  cfblk2 : Outport
  cfblk7 : Outport  Port=2
  wires:
  cfblk3/1 -> cfblk6/1(cfblk1)
  cfblk1/1 -> cfblk4/1
  cfblk6/1(cfblk2) -> cfblk5/1(cfblk1)
  cfblk6/2(cfblk8) -> cfblk7/1
  cfblk5/1(cfblk2) -> cfblk4/2
  cfblk6/3(cfblk9) -> cfblk5/2(cfblk12)
  cfblk6/4(cfblk10) -> cfblk2/1
  cfblk5/2(cfblk13) -> cfblk8/1
  cfblk8/1 -> cfblk6/2(cfblk6)
  cfblk5/3(cfblk14) -> cfblk9/1
  cfblk9/1 -> cfblk6/3(cfblk7)
  cfblk5/4(cfblk15) -> cfblk10/1
  cfblk10/1 -> cfblk3/1

== system sampleModel1000/cfblk153 ==
  cfblk1 : Inport
  cfblk7 : Inport  Port=2
  cfblk{10..13} (4 alike) : Delay  SampleTime=1
  cfblk3 : DiscreteFilter  SampleTime=1
  cfblk4 : Subsystem
  cfblk5 : Subsystem
  cfblk6 : If  IfExpression=u1 >= 0  SampleTime=1
  cfblk8 : Subsystem  TreatAsAtomicUnit=on
  cfblk9 : Subsystem  TreatAsAtomicUnit=on
  cfblk2 : Outport
  wires:
  cfblk7/1 -> cfblk8/1(cfblk1)
  cfblk1/1 -> cfblk6/1
  cfblk4/2(cfblk16) -> cfblk3/1
  cfblk8/1(cfblk2) -> cfblk9/3(cfblk15)
  cfblk4/3(cfblk17) -> cfblk5/1(cfblk1)
  cfblk8/2(cfblk11) -> cfblk2/1
  cfblk8/3(cfblk12) -> cfblk4/2(cfblk14)
  cfblk8/4(cfblk13) -> cfblk9/4(cfblk16)
  cfblk8/5(cfblk14) -> cfblk4/3(cfblk15)
  cfblk6/1 -> cfblk8/Action
  cfblk6/2 -> cfblk9/Action
  cfblk9/1(cfblk2) -> cfblk10/1
  cfblk10/1 -> cfblk8/2(cfblk10)
  cfblk4/1(cfblk2) -> cfblk11/1
  cfblk11/1 -> cfblk9/1(cfblk1)
  cfblk3/1 -> cfblk12/1
  cfblk12/1 -> cfblk4/1(cfblk1)
  cfblk5/1(cfblk2) -> cfblk13/1
  cfblk13/1 -> cfblk9/2(cfblk14)

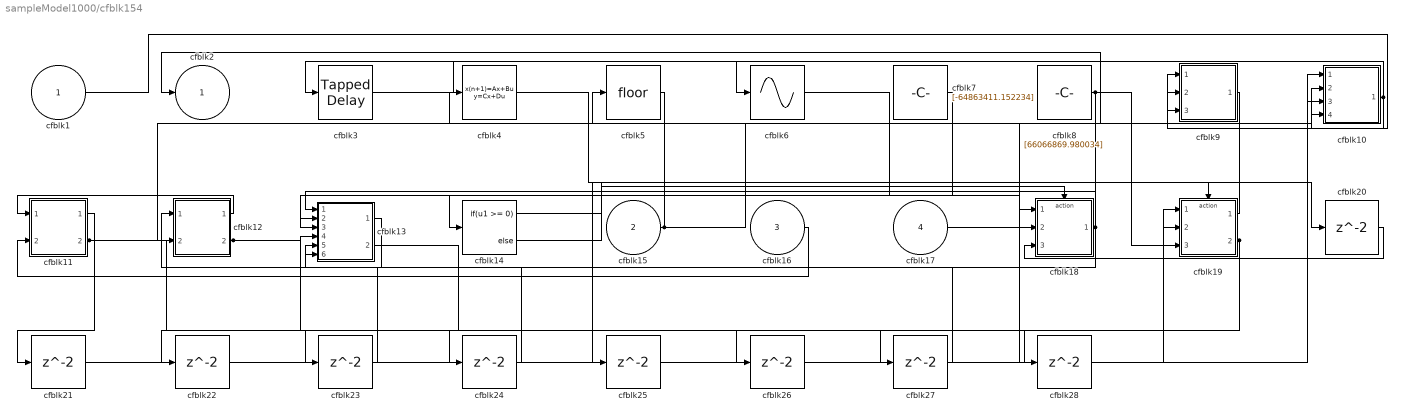
== system sampleModel1000/cfblk154 ==
  cfblk1 : Inport
  cfblk15 : Inport  Port=2
  cfblk16 : Inport  Port=3
  cfblk17 : Inport  Port=4
  cfblk10 : Subsystem
  cfblk11 : Subsystem
  cfblk12 : Subsystem
  cfblk13 : Subsystem
  cfblk14 : If  IfExpression=u1 >= 0  SampleTime=1
  cfblk18 : Subsystem  TreatAsAtomicUnit=on
  cfblk19 : Subsystem  TreatAsAtomicUnit=on
  cfblk{20..28} (9 alike) : Delay  SampleTime=1
  cfblk3 : simulink/Discrete/Tapped Delay  vinit=0.0  samptime=-1  NumDelays=1  DelayOrder=Oldest  includeCurrent=off
  cfblk4 : DiscreteStateSpace
  cfblk5 : Rounding
  cfblk6 : Sin  TimeSource=Use external signal  SampleTime=0
  cfblk7 : Constant  Value=[-64863411.152234]  SampleTime=1
  cfblk8 : Constant  Value=[66066869.980034]  SampleTime=1
  cfblk9 : Subsystem
  cfblk2 : Outport
  wires:
  cfblk8/1 -> cfblk13/1(cfblk1), cfblk19/3(cfblk9)
  cfblk7/1 -> cfblk14/1
  cfblk3/1 -> cfblk6/1
  cfblk19/1(cfblk2) -> cfblk2/1
  cfblk18/1(cfblk2) -> cfblk4/1, cfblk13/5(cfblk13)
  cfblk12/1(cfblk2) -> cfblk11/1(cfblk1)
  cfblk13/1(cfblk2) -> cfblk12/1(cfblk1)
  cfblk19/2(cfblk10) -> cfblk22/1, cfblk23/1
  cfblk12/2(cfblk14) -> cfblk26/1, cfblk27/1
  cfblk10/1(cfblk2) -> cfblk3/1, cfblk9/2(cfblk9)
  cfblk5/1 -> cfblk13/2(cfblk10)
  cfblk1/1 -> cfblk10/2(cfblk10)
  cfblk16/1 -> cfblk11/2(cfblk6)
  cfblk15/1 -> cfblk5/1, cfblk13/3(cfblk11), cfblk9/1(cfblk1)
  cfblk6/1 -> cfblk18/2(cfblk16)
  cfblk17/1 -> cfblk10/4(cfblk12)
  cfblk11/2(cfblk7) -> cfblk9/3(cfblk10), cfblk24/1
  cfblk14/1 -> cfblk18/Action
  cfblk14/2 -> cfblk19/Action
  cfblk4/1 -> cfblk20/1
  cfblk20/1 -> cfblk18/3(cfblk17)
  cfblk11/1(cfblk2) -> cfblk21/1
  cfblk21/1 -> cfblk19/2(cfblk8)
  cfblk22/1 -> cfblk18/1(cfblk1)
  cfblk23/1 -> cfblk13/4(cfblk12)
  cfblk24/1 -> cfblk12/2(cfblk13)
  cfblk9/1(cfblk2) -> cfblk25/1
  cfblk25/1 -> cfblk19/1(cfblk1)
  cfblk26/1 -> cfblk10/1(cfblk1)
  cfblk27/1 -> cfblk13/6(cfblk14)
  cfblk13/2(cfblk15) -> cfblk28/1
  cfblk28/1 -> cfblk10/3(cfblk11)

== system sampleModel1000/cfblk155 ==
  cfblk1 : Inport
  cfblk9 : Inport  Port=2
  cfblk{11..19} (9 alike) : Delay  SampleTime=1
  cfblk3 : Delay  DelayLengthSource=Input port  SampleTime=1
      settings: InputPortMap=u0,p1
  cfblk4 : Subsystem
  cfblk5 : Subsystem
  cfblk6 : Subsystem
  cfblk7 : Subsystem
  cfblk8 : Subsystem
  cfblk2 : Outport
  cfblk10 : Outport  Port=2
  wires:
  cfblk7/1(cfblk2) -> cfblk2/1, cfblk13/1, cfblk14/1, cfblk15/1
  cfblk3/1 -> cfblk10/1, cfblk6/3(cfblk13)
  cfblk9/1 -> cfblk6/1(cfblk1)
  cfblk5/1(cfblk2) -> cfblk3/1, cfblk8/3(cfblk10)
  cfblk6/2(cfblk14) -> cfblk8/1(cfblk1)
  cfblk4/1(cfblk2) -> cfblk7/1(cfblk1)
  cfblk8/2(cfblk13) -> cfblk4/1(cfblk1)
  cfblk1/1 -> cfblk5/3(cfblk10)
  cfblk6/3(cfblk15) -> cfblk4/2(cfblk11)
  cfblk4/3(cfblk14) -> cfblk17/1, cfblk18/1
  cfblk6/1(cfblk2) -> cfblk11/1
  cfblk11/1 -> cfblk5/2(cfblk9)
  cfblk8/1(cfblk2) -> cfblk12/1
  cfblk12/1 -> cfblk5/1(cfblk1)
  cfblk13/1 -> cfblk4/3(cfblk12)
  cfblk14/1 -> cfblk8/4(cfblk11)
  cfblk15/1 -> cfblk8/5(cfblk12)
  cfblk4/2(cfblk13) -> cfblk16/1
  cfblk16/1 -> cfblk8/2(cfblk9)
  cfblk17/1 -> cfblk6/2(cfblk12)
  cfblk18/1 -> cfblk5/4(cfblk11)
  cfblk6/4(cfblk16) -> cfblk19/1
  cfblk19/1 -> cfblk3/2

== system sampleModel1000/cfblk156 ==
  cfblk1 : Inport
  cfblk12 : Inport  Port=2
  cfblk10 : Subsystem
  cfblk11 : Subsystem
  cfblk3 : simulink/Discrete/Tapped Delay  vinit=0.0  samptime=-1  NumDelays=1  DelayOrder=Oldest  includeCurrent=off
  cfblk4 : simulink/Discrete/Difference  ICPrevInput=0.0  OutMin=[]  OutMax=[]  OutDataTypeStr=Inherit: Inherit via back propagation  OutDataType=fixdt(1, 16)  OutScaling=2^-10  DoSatur=off
  cfblk5 : Math  Operator=conj
  cfblk6 : Sum  Inputs=+-
  cfblk7 : Constant  Value=[-239733762.117171]  SampleTime=1
  cfblk8 : Constant  Value=[391630151.528436]  SampleTime=1
  cfblk9 : Subsystem
  cfblk2 : Outport
  cfblk13 : Outport  Port=2
  wires:
  cfblk12/1 -> cfblk11/1(cfblk1)
  cfblk11/1(cfblk2) -> cfblk13/1
  cfblk5/1 -> cfblk4/1, cfblk11/5(cfblk16), cfblk9/4(cfblk12)
  cfblk7/1 -> cfblk3/1, cfblk9/3(cfblk11)
  cfblk3/1 -> cfblk5/1, cfblk11/3(cfblk14), cfblk9/5(cfblk13)
  cfblk4/1 -> cfblk10/1(cfblk1)
  cfblk10/1(cfblk2) -> cfblk6/1
  cfblk6/1 -> cfblk2/1
  cfblk8/1 -> cfblk9/1(cfblk1), cfblk11/4(cfblk15)
  cfblk1/1 -> cfblk10/2(cfblk10), cfblk9/2(cfblk10)
  cfblk9/1(cfblk2) -> cfblk10/3(cfblk11)
  cfblk9/2(cfblk14) -> cfblk11/2(cfblk13), cfblk6/2

== system sampleModel1000/cfblk157 ==
  cfblk1 : Inport
  cfblk10 : Inport  Port=2
  cfblk{11..14} (4 alike) : Delay  SampleTime=1
  cfblk3 : DiscreteFir  SampleTime=1
  cfblk4 : Sum  Inputs=+-
  cfblk5 : Constant  Value=[-872505828.112506]  SampleTime=1
  cfblk6 : Constant  Value=[720630594.187512]  SampleTime=1
  cfblk7 : Subsystem
  cfblk8 : Subsystem
  cfblk9 : Subsystem
  cfblk2 : Outport
  wires:
  cfblk1/1 -> cfblk8/1(cfblk1), cfblk8/3(cfblk9), cfblk7/4(cfblk9), cfblk8/6(cfblk12)
  cfblk8/1(cfblk2) -> cfblk4/1
  cfblk10/1 -> cfblk9/1(cfblk1)
  cfblk7/1(cfblk2) -> cfblk11/1, cfblk12/1
  cfblk5/1 -> cfblk3/1
  cfblk6/1 -> cfblk2/1
  cfblk3/1 -> cfblk7/1(cfblk1)
  cfblk8/2(cfblk13) -> cfblk9/2(cfblk11)
  cfblk8/3(cfblk14) -> cfblk9/3(cfblk12)
  cfblk9/2(cfblk13) -> cfblk7/2(cfblk7), cfblk14/1
  cfblk4/1 -> cfblk7/3(cfblk8)
  cfblk11/1 -> cfblk4/2
  cfblk12/1 -> cfblk8/4(cfblk10)
  cfblk9/1(cfblk2) -> cfblk13/1
  cfblk13/1 -> cfblk8/2(cfblk8)
  cfblk14/1 -> cfblk8/5(cfblk11)

== system sampleModel1000/cfblk158 ==
  cfblk1 : Inport
  cfblk8 : Inport  Port=2
  cfblk10 : Delay  SampleTime=1
  cfblk3 : Delay  SampleTime=1
  cfblk4 : UnaryMinus
  cfblk5 : Subsystem
  cfblk6 : Subsystem
  cfblk7 : Subsystem
  cfblk9 : Delay  SampleTime=1
  cfblk2 : Outport
  wires:
  cfblk5/1(cfblk2) -> cfblk2/1
  cfblk3/1 -> cfblk5/1(cfblk1), cfblk5/3(cfblk15), cfblk9/1
  cfblk7/1(cfblk2) -> cfblk3/1, cfblk10/1
  cfblk8/1 -> cfblk7/2(cfblk12), cfblk5/2(cfblk14)
  cfblk6/1(cfblk2) -> cfblk7/3(cfblk13), cfblk5/4(cfblk16)
  cfblk1/1 -> cfblk4/1, cfblk6/2(cfblk12)
  cfblk4/1 -> cfblk6/1(cfblk1)
  cfblk9/1 -> cfblk7/1(cfblk1)
  cfblk10/1 -> cfblk6/3(cfblk13)

== system sampleModel1000/cfblk159 ==
  cfblk1 : Inport
  cfblk14 : Inport  Port=2
  cfblk15 : Inport  Port=3
  cfblk10 : Subsystem
  cfblk11 : Subsystem
  cfblk12 : Subsystem
  cfblk13 : Subsystem
  cfblk16 : Delay  SampleTime=1
  cfblk17 : Delay  SampleTime=1
  cfblk3 : simulink/Discrete/Difference  ICPrevInput=0.0  OutMin=[]  OutMax=[]  OutDataTypeStr=Inherit: Inherit via back propagation  OutDataType=fixdt(1, 16)  OutScaling=2^-10  DoSatur=off
  cfblk4 : DiscreteIntegrator  ICPrevOutput=DiscIntNeverNeededParam  ICPrevScaledInput=DiscIntNeverNeededParam
  cfblk5 : simulink/Discrete/Tapped Delay  vinit=0.0  samptime=-1  NumDelays=1  DelayOrder=Oldest  includeCurrent=off
  cfblk6 : Sqrt  Operator=rSqrt  AlgorithmType=Newton-Raphson
  cfblk7 : Constant  Value=[900135045.430387]  SampleTime=1
  cfblk8 : Constant  Value=[139090620.927687]  SampleTime=1
  cfblk9 : Subsystem
  cfblk2 : Outport
  wires:
  cfblk1/1 -> cfblk11/1(cfblk1)
  cfblk4/1 -> cfblk13/1(cfblk1)
  cfblk7/1 -> cfblk3/1
  cfblk5/1 -> cfblk10/1(cfblk1)
  cfblk15/1 -> cfblk4/1
  cfblk6/1 -> cfblk5/1
  cfblk12/1(cfblk2) -> cfblk9/1(cfblk1)
  cfblk3/1 -> cfblk13/2(cfblk14)
  cfblk8/1 -> cfblk12/1(cfblk1)
  cfblk12/2(cfblk17) -> cfblk6/1
  cfblk13/1(cfblk2) -> cfblk2/1
  cfblk14/1 -> cfblk11/2(cfblk11)
  cfblk11/1(cfblk2) -> cfblk12/3(cfblk15)
  cfblk13/2(cfblk15) -> cfblk12/4(cfblk16)
  cfblk9/1(cfblk2) -> cfblk16/1
  cfblk16/1 -> cfblk12/2(cfblk14)
  cfblk10/1(cfblk2) -> cfblk17/1
  cfblk17/1 -> cfblk11/3(cfblk12)

== system sampleModel1000/cfblk160 ==
  cfblk1 : Inport
  cfblk3 : DiscreteStateSpace
  cfblk4 : simulink/Discrete/Tapped Delay  vinit=0.0  samptime=-1  NumDelays=1  DelayOrder=Oldest  includeCurrent=off
  cfblk5 : Sum  Inputs=+
  cfblk6 : Sum  Inputs=+
  cfblk7 : Constant  Value=[684150714.597674]  SampleTime=1
  cfblk2 : Outport
  wires:
  cfblk5/1 -> cfblk4/1
  cfblk7/1 -> cfblk5/1
  cfblk6/1 -> cfblk3/1
  cfblk3/1 -> cfblk2/1
  cfblk1/1 -> cfblk6/1

== system sampleModel1000/cfblk161 ==
  cfblk1 : Inport
  cfblk10 : If  IfExpression=u1 >= 0  SampleTime=1
  cfblk11 : Subsystem  TreatAsAtomicUnit=on
  cfblk12 : Subsystem  TreatAsAtomicUnit=on
  cfblk{13..19} (7 alike) : Delay  SampleTime=1
  cfblk3 : simulink/Discrete/Tapped Delay  vinit=0.0  samptime=-1  NumDelays=1  DelayOrder=Oldest  includeCurrent=off
  cfblk4 : DiscreteStateSpace
  cfblk5 : ComplexToMagnitudeAngle
  cfblk6 : Constant  Value=[-245586379.071807]  SampleTime=1
  cfblk7 : Subsystem
  cfblk8 : Subsystem
  cfblk9 : Subsystem
  cfblk2 : Outport
  wires:
  cfblk8/1(cfblk2) -> cfblk9/3(cfblk11), cfblk13/1
  cfblk11/1(cfblk2) -> cfblk2/1
  cfblk6/1 -> cfblk11/2(cfblk12)
  cfblk12/1(cfblk2) -> cfblk3/1, cfblk16/1
  cfblk9/1(cfblk2) -> cfblk4/1
  cfblk11/2(cfblk14) -> cfblk7/1(cfblk1)
  cfblk5/1 -> cfblk10/1
  cfblk1/1 -> cfblk5/1
  cfblk5/2 -> cfblk11/3(cfblk13), cfblk9/7(cfblk15)
  cfblk9/2(cfblk16) -> cfblk17/1, cfblk18/1
  cfblk11/3(cfblk15) -> cfblk7/2(cfblk13), cfblk9/4(cfblk12)
  cfblk7/1(cfblk2) -> cfblk8/2(cfblk8)
  cfblk7/3(cfblk17) -> cfblk8/3(cfblk9), cfblk9/1(cfblk1), cfblk9/2(cfblk10), cfblk9/5(cfblk13), cfblk9/6(cfblk14)
  cfblk10/1 -> cfblk11/Action
  cfblk10/2 -> cfblk12/Action
  cfblk13/1 -> cfblk11/1(cfblk1)
  cfblk4/1 -> cfblk14/1
  cfblk14/1 -> cfblk12/1(cfblk1)
  cfblk3/1 -> cfblk15/1
  cfblk15/1 -> cfblk8/1(cfblk1)
  cfblk16/1 -> cfblk7/4(cfblk15)
  cfblk17/1 -> cfblk12/2(cfblk12)
  cfblk18/1 -> cfblk7/3(cfblk14)
  cfblk7/2(cfblk16) -> cfblk19/1
  cfblk19/1 -> cfblk12/3(cfblk13)
